simulink model "airconditioner"  (R2024b)
settings: Solver=VariableStepAuto  StartTime=0.0  StopTime=10.0  RelTol=1e-3
settings Model: Creator=sushm  LastModifiedBy=sushm

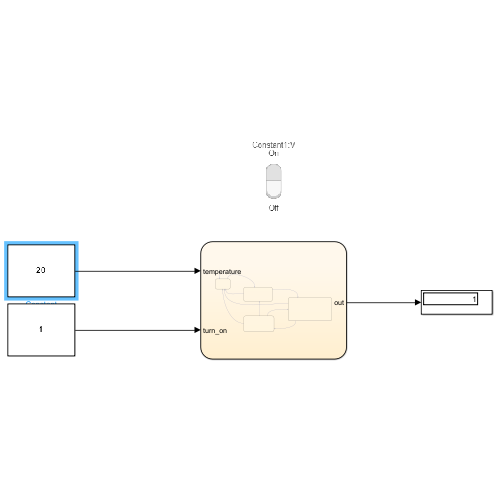
[thumbnail: Simulink's stored preview of the top-level diagram]
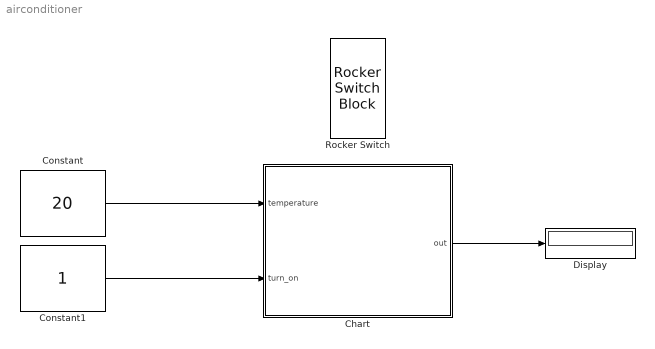
== system airconditioner ==
  Chart : Stateflow chart  TreatAsAtomicUnit=on
  Constant : Constant  Value=20
  Constant1 : Constant
  Display : Display
  Rocker Switch : RockerSwitchBlock
      settings: Values={{'Off', 'On'}, [0 1]}
  wires:
  Constant/1 -> Chart/1(temperature)
  Constant1/1 -> Chart/2(turn_on)
  Chart/1(out) -> Display/1

== stateflow chart airconditioner/Chart ==
  state on_off
    out=0
  state steady
    out=heat_temp
  state heat_on
    heat_temp=heat_temp+1
    out=heat_temp
  state cooler_on
    heat_temp=heat_temp-1
    out=heat_temp
  (default) -> on_off : {heat_temp=0}
  on_off -> state3 : [turn_on==1]
  cooler_on -> on_off [order 2] : [turn_on==0]
  heat_on -> on_off [order 2] : [turn_on==0]
  state3 -> on_off [order 2] : [turn_on==0]
  state3 -> heat_on [order 1] : [turn_on==1&&...
      | heat_temp<temperature]
  cooler_on -> state3 [order 3] : [turn_on==1&&...
      | heat_temp==temperature]
  cooler_on -> heat_on [order 1] : [heat_temp<temperature]
  heat_on -> cooler_on [order 1] : [heat_temp>temperature]
  data: temperature input; heat_temp local; out output; turn_on input
